simulink model "nonlinear_Plant"  (Simulink 8.1)
settings: Solver=ode45  StartTime=0.0  StopTime=10000  FixedStep=0.001  RelTol=1e-3
values from neighbouring files (symbols this model uses):
  a_m = -4    [MRAC_script.m]
  a_p = 1    [MRAC_script.m]
  Gamma = eye(6)*2    [MRAC_script.m]
  k_m = 4    [MRAC_script.m]
  k_p = 3    [MRAC_script.m]
  k_star = k_m/k_p    (= 1.33333333333)    [MRAC_script.m]
  param_0 = [0 0 0 0 0 0]    [MRAC_script.m]
  theta_f = [0 -1 1 0]    [MRAC_script.m]
  theta_star = (a_m-a_p)/k_p    (= -1.66666666667)    [MRAC_script.m]
  x_m_0 = 0    [MRAC_script.m]
  x_p_0 = 0    [MRAC_script.m]
settings Model: Creator=patrick  LastModifiedBy=patrick
settings DataIOCC: SignalLoggingSaveFormat=Dataset
settings OptimizationCC: ExpressionDepthLimit=128
settings DebuggingCC: UnderspecifiedInitializationDetection=Simplified  FcnCallInpInsideContextMsg=EnableAllAsError  StateNameClashWarn=none
settings GRTTargetCC: CodeReplacementLibrary=C89/C90 (ANSI)  CombineOutputUpdateFcns=on  GRTInterface=off

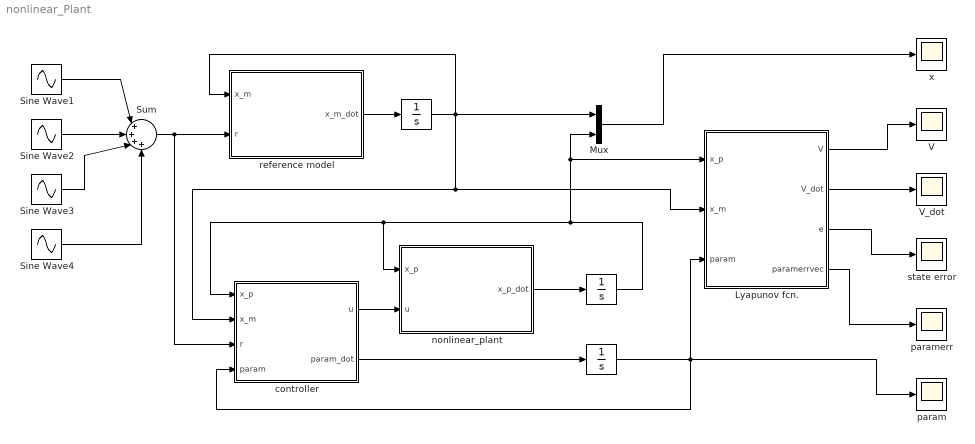
== system nonlinear_Plant ==
  " " : Integrator  InitialCondition=param_0
  "    " : Integrator  InitialCondition=x_p_0
  "                  " : Integrator  InitialCondition=x_m_0
  Lyapunov fcn. : MATLAB Function  TreatAsAtomicUnit=on
      settings: PermitHierarchicalResolution=ParametersOnly
  Mux : Mux  Inputs=2
  Sine Wave1 : Sin  Frequency=3  SampleTime=0
  Sine Wave2 : Sin  Frequency=3/2  SampleTime=0
  Sine Wave3 : Sin  Frequency=3/4  SampleTime=0
  Sine Wave4 : Sin  Frequency=3/8  SampleTime=0
  Sum : Sum  Inputs=|++++
  V : Scope
      settings: SaveName=lyapunov
  V_dot : Scope
      settings: SaveName=lyapunov_dot
  controller : MATLAB Function  TreatAsAtomicUnit=on
      settings: PermitHierarchicalResolution=ParametersOnly
  nonlinear_plant : MATLAB Function  TreatAsAtomicUnit=on
      settings: PermitHierarchicalResolution=ParametersOnly
  param : Scope
      settings: SaveName=parameters
  paramerr : Scope
      settings: SaveName=parameter_errors
  reference model : MATLAB Function  TreatAsAtomicUnit=on
      settings: PermitHierarchicalResolution=ParametersOnly
  state error : Scope
      settings: YMin=-0.225  YMax=0.3  SaveName=error
  "x " : Scope
      settings: SaveName=modelAndPlant
  wires:
  controller/1(u) -> nonlinear_plant/2(u)
  reference model/1(x_m_dot) -> "                  "/1
  nonlinear_plant/1(x_p_dot) -> "    "/1
  "    "/1 -> nonlinear_plant/1(x_p), controller/1(x_p), Lyapunov fcn./1(x_p), Mux/2
  "                  "/1 -> reference model/1(x_m), Mux/1, controller/2(x_m), Lyapunov fcn./2(x_m)
  controller/2(param_dot) -> " "/1
  Mux/1 -> "x "/1
  Sum/1 -> controller/3(r), reference model/2(r)
  Lyapunov fcn./1(V) -> V/1
  Lyapunov fcn./2(V_dot) -> V_dot/1
  Sine Wave1/1 -> Sum/1
  Sine Wave2/1 -> Sum/2
  Sine Wave3/1 -> Sum/3
  Sine Wave4/1 -> Sum/4
  Lyapunov fcn./4(paramerrvec) -> paramerr/1
  " "/1 -> Lyapunov fcn./3(param), param/1, controller/4(param)
  Lyapunov fcn./3(e) -> state error/1

== matlab function reference model ==
  data: x_m_dot output double; x_m input double; r input double; a_m parameter double; k_m parameter double
function x_m_dot = reference_model(x_m, r, a_m, k_m)

x_m_dot=a_m*x_m+k_m*r;      %reference model dynamics with parameters from script

end

== matlab function controller ==
  data: u output double; x_p input double; k_p parameter double; x_m input double; r input double; param input double; Gamma parameter double; param_dot output double
function [u, param_dot] = controller(x_p, k_p, x_m, r, param, Gamma)

e=x_p-x_m;                                                                 %state error

Phi_f=[x_p^3; exp(-10*(x_p+0.5)^2); exp(-10*(x_p-0.5)^2); sin(2*x_p)];     %structure of the nonlinearyties

regressor=[x_p; r; Phi_f];                                                 %regressor vector

param_dot=-sign(k_p)*Gamma*regressor*e;                                    %adaptive law

u=param'*regressor;                                                        %control signal

end

== matlab function nonlinear_plant ==
  data: x_p_dot output double; x_p input double; a_p parameter double; k_p parameter double; u input double; theta_f parameter double
function x_p_dot = plant(x_p, a_p, k_p, u, theta_f)

f=theta_f*[x_p^3; exp(-10*(x_p+0.5)^2); exp(-10*(x_p-0.5)^2); sin(2*x_p)];   %nonlinear function

x_p_dot=a_p*x_p+k_p*u-k_p*f;                                                 %plant dynamics with nonlinear part

end

== matlab function Lyapunov fcn. ==
  data: V output double; x_p input double; x_m input double; k_p parameter double; a_m parameter double; param input double; theta_star parameter double; k_star parameter double; V_dot output double; e output double; theta_f parameter double; Gamma parameter double; paramerrvec output double
function [V, V_dot, e, paramerrvec] = lyapunov_fcn(x_p, x_m,k_p, a_m, param, theta_star, k_star, theta_f, Gamma)

e=x_p-x_m;                                                      %state error

param_star=[theta_star, k_star, theta_f];                       %true parameters red from script stored in vector

paramerrvec=param-param_star';                                  %parameter errorvector

V=0.5*e^2+0.5*abs(k_p)*(paramerrvec'*Gamma^(-1)*paramerrvec);   %Lyapunov function

V_dot=a_m*e^2;                                                  %Lyapunov function derrivative

end
